simulink model "ME655_Lect09_VL3_Simulink"  (R2021b)
settings: Solver=FixedStepAuto  StartTime=0.0  StopTime=60.0  FixedStep=.003  RelTol=1e-3
values from neighbouring files (symbols this model uses):
  dt_active_control = 10    [ME655_Lect09_VL3_MATLAB.m]
  h = 2.5*N    (= 200)    [ME655_Lect09_VL3_MATLAB.m]
  lambda = .95    (= 0.95)    [ME655_Lect09_VL3_MATLAB.m]
  Lhip_pos0 = Lhip_pos(1)    [ME655_Lect09_VL3_MATLAB.m]
  Lhip_vel0 = Lhip_vel(1)    [ME655_Lect09_VL3_MATLAB.m]
  M = 6    [ME655_Lect09_VL3_MATLAB.m]
  N = 80    [ME655_Lect09_VL3_MATLAB.m]
  nu = .5    (= 0.5)    [ME655_Lect09_VL3_MATLAB.m]
  t_start = 5.0    (= 5)    [ME655_Lect09_VL3_MATLAB.m]
  Tau_h_max = 30    [ME655_Lect09_VL3_MATLAB.m]
undefined symbols (not defined in the file or in its folder): Bh, g, IHC, IRC, Kh, LH, LR, mH, mR, theta_0, theta_d0
settings Model: Creator=Damiano  LastModifiedBy=ilanazane
settings SolverCC: AlgebraicLoopSolver=TrustRegion
settings DataIOCC: ReturnWorkspaceOutputs=off
settings DebuggingCC: SFMachineParentedDataDiag=warning  ArithmeticOperatorsInVariantConditions=warning
settings SFSimCC: SimUseLocalCustomCode=off  CustomCodeUndefinedFunction=UseInterfaceOnly
settings RTWCC: RTWUseLocalCustomCode=off
settings CodeAppCC: StateflowObjectComments=on

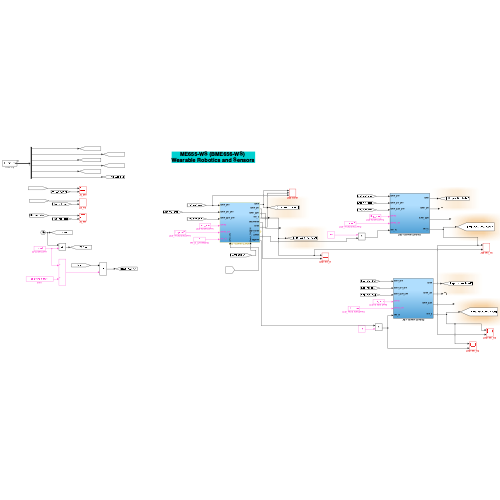
[thumbnail: Simulink's stored preview of the top-level diagram]
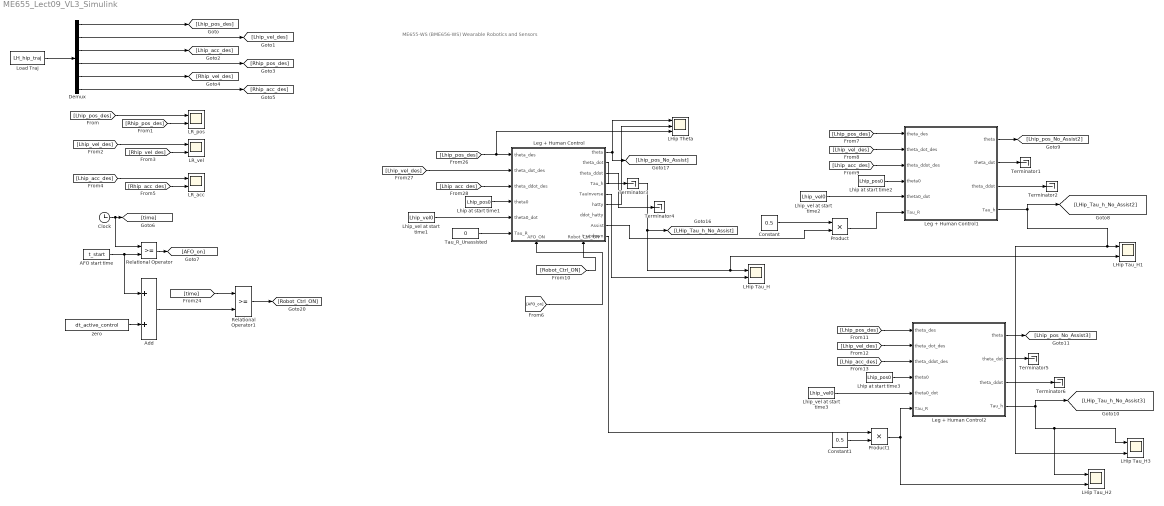
== system ME655_Lect09_VL3_Simulink ==
  note: ME655-WS (BME656-WS)
      | Wearable Robotics and Sensors
  AFO start time : Constant  Value=t_start
  Add : Sum
  Clock : Clock
  Constant : Constant  Value=0.5
  Constant1 : Constant  Value=0.5
  Demux : Demux  Outputs=6
  LHip Tau_H{,1..3} (4 alike) : Scope  NumInputPorts=2
  LHip Theta : Scope  NumInputPorts=3
  "LR_acc " : Scope  NumInputPorts=2
  LR_pos : Scope  NumInputPorts=2
  LR_vel : Scope  NumInputPorts=2
  Leg + Human Control : Subsystem
      settings: PortSchema="{\"entries\":[{\"content\":{\"sides\":[{\"content\":{\"connectorIds\":[\"In1\",\"In2\",\"In3\",\"In4\",\"In5\",\"In6\"]},\"type\":\"ConnectorPlacement.EquallySpacedRectSide\",\"uuid\":\"c89990dd-c7dc-4056-83f4-5e6c1198dd9e\"},{\"content\":{\"connectorIds\":[\"Out1\",\"Out2\",\"Out3\",\"Out4\",\"Out5\",\"Out6\",\"Out7\",\"Out8\",\"Out9\"],\"side\":\"RIGHT\"},\"type\":\"ConnectorPlacement.EquallySpacedRectSide\",\"uuid\":\"97852725-6742-4674-9802-faa7978f5241\"},{\"content\":{\"connectorIds\":[],\"side\":\"TOP\"},\"type\":\"ConnectorPlacement.EquallySpacedRectSide\",\"uuid\":\"eb4c760c-f7ff-400d-9b3e-843f42fb2cfa\"},{\"content\":{\"connectorIds\":[\"In7\",\"In8\"],\"side\":\"BOTTOM\"},\"type\":\"ConnectorPlacement.EquallySpacedRectSide\",\"uuid\":\"cb588bf4-9441-43b4-ae6d-1958c203e45c\"}]},\"type\":\"ConnectorPlacement.EquallySpacedConnector\",\"uuid\":\"443be17b-8f0d-444a-9eaa-10dcd6d34b91\"}],\"packageUris\":[\"http://schema.mathworks.com/mf0/Connector/R2020b\"],\"version\":\"1.0\"}"
  Leg + Human Control1 : Subsystem
  Leg + Human Control2 : Subsystem
  Lhip at start time1 : Constant  Value=Lhip_pos0
  Lhip at start time2 : Constant  Value=Lhip_pos0
  Lhip at start time3 : Constant  Value=Lhip_pos0
  Lhip_vel at start time1 : Constant  Value=Lhip_vel0
  Lhip_vel at start time2 : Constant  Value=Lhip_vel0
  Lhip_vel at start time3 : Constant  Value=Lhip_vel0
  Load Traj : FromWorkspace  VariableName=LH_hip_traj
  Product : Product
  Product1 : Product
  Relational Operator : RelationalOperator  OutDataTypeStr=boolean  RndMeth=Simplest
  Relational Operator1 : RelationalOperator  OutDataTypeStr=boolean  RndMeth=Simplest
  Tau_R_Unassisted : Constant  Value=0
  Terminator{1..6} (6 alike) : Terminator
  zero : Constant  Value=dt_active_control
  wires:
  Load Traj/1 -> Demux/1
  Demux/6 -> [Rhip_acc_des]
  Demux/4 -> [Rhip_pos_des]
  Demux/5 -> [Rhip_vel_des]
  [Lhip_pos_des] -> LR_pos/1
  [Rhip_pos_des] -> LR_pos/2
  [Lhip_vel_des] -> LR_vel/1
  [Rhip_vel_des] -> LR_vel/2
  [Lhip_acc_des] -> "LR_acc "/1
  [Rhip_acc_des] -> "LR_acc "/2
  Clock/1 -> Relational Operator/1, [time]
  Relational Operator/1 -> [AFO_on]
  [time] -> Relational Operator1/1
  AFO start time/1 -> Add/1, Relational Operator/2
  Add/1 -> Relational Operator1/2
  zero/1 -> Add/2
  [Lhip_acc_des] -> Leg + Human Control/3(theta_ddot_des)
  Leg + Human Control/3(theta_ddot) -> Terminator4/1
  Lhip_vel at start time1/1 -> Leg + Human Control/5(theta0_dot)
  Leg + Human Control/2(theta_dot) -> Terminator3/1
  [Lhip_vel_des] -> Leg + Human Control/2(theta_dot_des)
  Lhip at start time1/1 -> Leg + Human Control/4(theta0)
  Leg + Human Control/1(theta) -> [Lhip_pos_No_Assist], LHip Theta/1
  Leg + Human Control/4(Tau_h) -> LHip Tau_H1/2, LHip Tau_H/1, [LHip_Tau_h_No_Assist]
  [Lhip_pos_des] -> Leg + Human Control/1(theta_des), LHip Theta/3
  Relational Operator1/1 -> [Robot_Ctrl_ON]
  Demux/1 -> [Lhip_pos_des]
  Demux/2 -> [Lhip_vel_des]
  Demux/3 -> [Lhip_acc_des]
  Leg + Human Control/5(TauInverse) -> LHip Tau_H/2
  Leg + Human Control/6(hatty) -> LHip Theta/2
  [AFO_on] -> Leg + Human Control/7(AFO_ON)
  Leg + Human Control1/4(Tau_h) -> LHip Tau_H3/2, LHip Tau_H1/1, [LHip_Tau_h_No_Assist2]
  [Lhip_pos_des] -> Leg + Human Control1/1(theta_des)
  Leg + Human Control1/2(theta_dot) -> Terminator1/1
  Lhip_vel at start time2/1 -> Leg + Human Control1/5(theta0_dot)
  [Lhip_acc_des] -> Leg + Human Control1/3(theta_ddot_des)
  Lhip at start time2/1 -> Leg + Human Control1/4(theta0)
  [Lhip_vel_des] -> Leg + Human Control1/2(theta_dot_des)
  Leg + Human Control1/1(theta) -> [Lhip_pos_No_Assist2]
  Leg + Human Control1/3(theta_ddot) -> Terminator2/1
  Tau_R_Unassisted/1 -> Leg + Human Control/6(Tau_R)
  Leg + Human Control/8(Assist) -> Product/2
  Constant/1 -> Product/1
  [Robot_Ctrl_ON] -> Leg + Human Control/8(Robot_Ctrl_ON)
  Product/1 -> Leg + Human Control1/6(Tau_R)
  [Lhip_pos_des] -> Leg + Human Control2/1(theta_des)
  Leg + Human Control2/4(Tau_h) -> LHip Tau_H2/1, LHip Tau_H3/1, [LHip_Tau_h_No_Assist3]
  Leg + Human Control2/1(theta) -> [Lhip_pos_No_Assist3]
  Lhip at start time3/1 -> Leg + Human Control2/4(theta0)
  Lhip_vel at start time3/1 -> Leg + Human Control2/5(theta0_dot)
  [Lhip_acc_des] -> Leg + Human Control2/3(theta_ddot_des)
  Leg + Human Control2/3(theta_ddot) -> Terminator6/1
  [Lhip_vel_des] -> Leg + Human Control2/2(theta_dot_des)
  Leg + Human Control2/2(theta_dot) -> Terminator5/1
  Leg + Human Control/9(t_updown) -> Product1/1
  Constant1/1 -> Product1/2
  Product1/1 -> LHip Tau_H2/2, Leg + Human Control2/6(Tau_R)

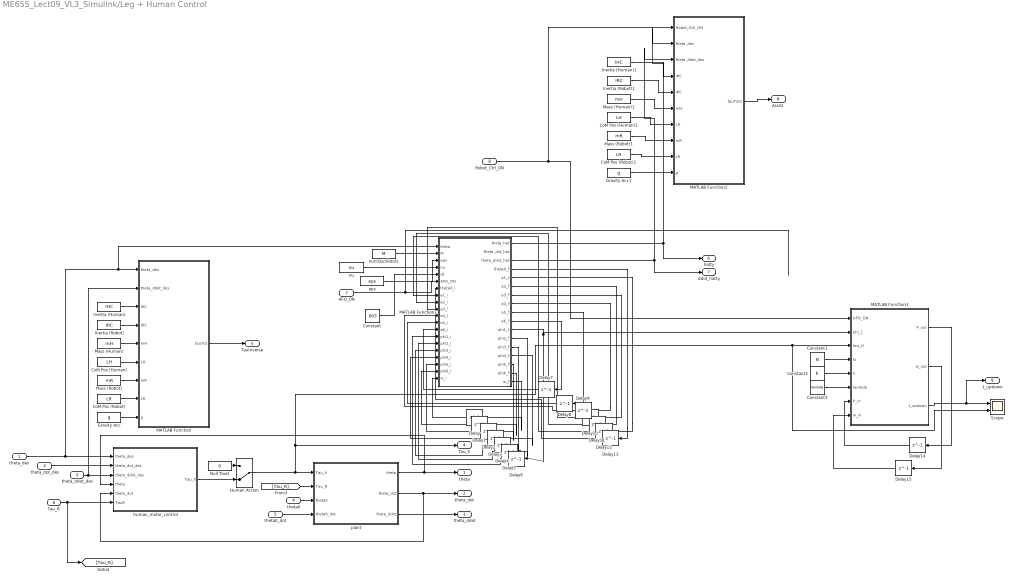
== system ME655_Lect09_VL3_Simulink/Leg + Human Control ==
  theta_des : Inport
  theta_dot_des : Inport  Port=2
  theta_ddot_des : Inport  Port=3
  theta0 : Inport  Port=4
  theta0_dot : Inport  Port=5
  Tau_R : Inport  Port=6
  AFO_ON : Inport  Port=7
  Robot_Ctrl_ON : Inport  Port=8
  CoM Pos (Human) : Constant  Value=LH
  CoM Pos (Human)1 : Constant  Value=LH
  CoM Pos (Robot) : Constant  Value=LR
  CoM Pos (Robot)1 : Constant  Value=LR
  Constant : Constant  Value=.003
  Constant1 : Constant  Value=N
  Constant2 : Constant  Value=h
  Constant3 : Constant  Value=lambda
  Delay{,1..15} (16 alike) : Delay  DelayLength=1  InitialCondition=0
  Gravity Acc : Constant  Value=g
  Gravity Acc1 : Constant  Value=g
  Human Action : ManualSwitch  CurrentSetting=0
  Inertia (Human) : Constant  Value=IHC
  Inertia (Human)1 : Constant  Value=IHC
  Inertia (Robot) : Constant  Value=IRC
  Inertia (Robot)1 : Constant  Value=IRC
  MATLAB Function : MATLAB Function  TreatAsAtomicUnit=on
  MATLAB Function1 : MATLAB Function  TreatAsAtomicUnit=on
  MATLAB Function2 : MATLAB Function  TreatAsAtomicUnit=on
  MATLAB Function3 : MATLAB Function  TreatAsAtomicUnit=on
  Mass (Human) : Constant  Value=mH
  Mass (Human)1 : Constant  Value=mH
  Mass (Robot) : Constant  Value=mR
  Mass (Robot)1 : Constant  Value=mR
  Null TauH : Constant  Value=0
  Scope : Scope  NumInputPorts=2
  eps : Constant  Value=eps
  human_motor_control : Subsystem
  nu : Constant  Value=nu
  numOscillators : Constant  Value=M
  plant : Subsystem
  theta : Outport  PortDimensions=[1,1]  VectorParamsAs1DForOutWhenUnconnected=off
  theta_dot : Outport  Port=2  PortDimensions=[1,1]  VectorParamsAs1DForOutWhenUnconnected=off
  theta_ddot : Outport  Port=3  PortDimensions=[1,1]  VectorParamsAs1DForOutWhenUnconnected=off
  Tau_h : Outport  Port=4  PortDimensions=[1,1]  VectorParamsAs1DForOutWhenUnconnected=off
  TauInverse : Outport  Port=5
  hatty : Outport  Port=6
  ddot_hatty : Outport  Port=7
  Assist : Outport  Port=8
  t_updown : Outport  Port=9
  wires:
  theta_des/1 -> MATLAB Function1/1(theta), MATLAB Function/1(theta_des), human_motor_control/1(theta_des)
  theta_dot_des/1 -> human_motor_control/2(theta_dot_des)
  theta0/1 -> plant/3(theta0)
  theta0_dot/1 -> plant/4(theta0_dot)
  [Tau_R] -> plant/2(Tau_R)
  plant/1(theta) -> theta/1, human_motor_control/4(theta)
  plant/2(theta_dot) -> human_motor_control/5(theta_dot), theta_dot/1
  plant/3(theta_ddot) -> theta_ddot/1
  theta_ddot_des/1 -> MATLAB Function/2(theta_ddot_des), human_motor_control/3(theta_ddot_des)
  human_motor_control/1(Tau_h) -> Human Action/2
  Human Action/1 -> Scope/2, MATLAB Function3/3(tau_H), Tau_h/1, plant/1(Tau_h)
  Null TauH/1 -> Human Action/1
  Tau_R/1 -> [Tau_R], human_motor_control/6(TauR)
  Inertia (Human)/1 -> MATLAB Function/3(IHC)
  Inertia (Robot)/1 -> MATLAB Function/4(IRC)
  Mass (Human)/1 -> MATLAB Function/5(mH)
  CoM Pos (Human)/1 -> MATLAB Function/6(LH)
  Mass (Robot)/1 -> MATLAB Function/7(mR)
  CoM Pos (Robot)/1 -> MATLAB Function/8(LR)
  Gravity Acc/1 -> MATLAB Function/9(g)
  MATLAB Function/1(tauTot) -> TauInverse/1
  numOscillators/1 -> MATLAB Function1/2(M)
  eps/1 -> MATLAB Function1/3(eps)
  nu/1 -> MATLAB Function1/4(nu)
  MATLAB Function1/17(w_f) -> Delay/1
  Delay/1 -> MATLAB Function1/20(w_i)
  MATLAB Function1/16(phi6_f) -> Delay1/1
  Delay1/1 -> MATLAB Function1/19(phi6_i)
  MATLAB Function1/15(phi5_f) -> Delay2/1
  Delay2/1 -> MATLAB Function1/18(phi5_i)
  MATLAB Function1/14(phi4_f) -> Delay3/1
  Delay3/1 -> MATLAB Function1/17(phi4_i)
  MATLAB Function1/13(phi3_f) -> Delay4/1
  Delay4/1 -> MATLAB Function1/16(phi3_i)
  MATLAB Function1/12(phi2_f) -> Delay5/1
  Delay5/1 -> MATLAB Function1/15(phi2_i)
  MATLAB Function1/11(phi1_f) -> Delay6/1, MATLAB Function3/2(phi_1)
  Delay6/1 -> MATLAB Function1/14(phi1_i)
  MATLAB Function1/10(a6_f) -> Delay7/1
  Delay7/1 -> MATLAB Function1/13(a6_i)
  MATLAB Function1/9(a5_f) -> Delay8/1
  Delay8/1 -> MATLAB Function1/12(a5_i)
  MATLAB Function1/8(a4_f) -> Delay9/1
  Delay9/1 -> MATLAB Function1/11(a4_i)
  MATLAB Function1/7(a3_f) -> Delay10/1
  Delay10/1 -> MATLAB Function1/10(a3_i)
  MATLAB Function1/6(a2_f) -> Delay11/1
  Delay11/1 -> MATLAB Function1/9(a2_i)
  MATLAB Function1/5(a1_f) -> Delay12/1
  Delay12/1 -> MATLAB Function1/8(a1_i)
  MATLAB Function1/4(theta0_f) -> Delay13/1
  Delay13/1 -> MATLAB Function1/7(theta0_i)
  Constant/1 -> MATLAB Function1/5(dt)
  MATLAB Function1/1(theta_hat) -> MATLAB Function2/2(theta_des), hatty/1
  AFO_ON/1 -> MATLAB Function1/6(AFO_ON)
  MATLAB Function1/3(theta_ddot_hat) -> ddot_hatty/1, MATLAB Function2/3(theta_ddot_des)
  Inertia (Human)1/1 -> MATLAB Function2/4(IHC)
  Inertia (Robot)1/1 -> MATLAB Function2/5(IRC)
  Mass (Human)1/1 -> MATLAB Function2/6(mH)
  CoM Pos (Human)1/1 -> MATLAB Function2/7(LH)
  Mass (Robot)1/1 -> MATLAB Function2/8(mR)
  CoM Pos (Robot)1/1 -> MATLAB Function2/9(LR)
  Gravity Acc1/1 -> MATLAB Function2/10(g)
  MATLAB Function2/1(tauTot2) -> Assist/1
  Robot_Ctrl_ON/1 -> MATLAB Function3/1(AFO_ON), MATLAB Function2/1(Robot_Ctrl_ON)
  Constant1/1 -> MATLAB Function3/4(N)
  Constant2/1 -> MATLAB Function3/5(h)
  Constant3/1 -> MATLAB Function3/6(lambda)
  Delay14/1 -> MATLAB Function3/7(P_in)
  MATLAB Function3/1(P_out) -> Delay14/1
  MATLAB Function3/2(w_out) -> Delay15/1
  Delay15/1 -> MATLAB Function3/8(w_in)
  MATLAB Function3/3(t_updown) -> t_updown/1, Scope/1

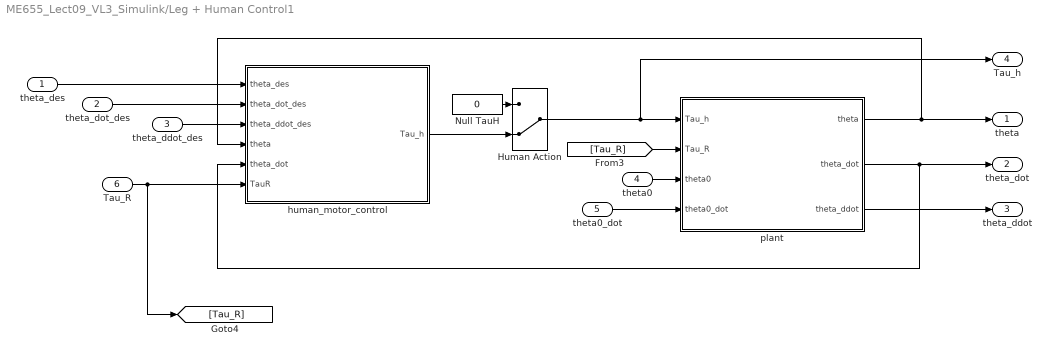
== system ME655_Lect09_VL3_Simulink/Leg + Human Control1 ==
  theta_des : Inport
  theta_dot_des : Inport  Port=2
  theta_ddot_des : Inport  Port=3
  theta0 : Inport  Port=4
  theta0_dot : Inport  Port=5
  Tau_R : Inport  Port=6
  Human Action : ManualSwitch  CurrentSetting=0
  Null TauH : Constant  Value=0
  human_motor_control : Subsystem
  plant : Subsystem
  theta : Outport  PortDimensions=[1,1]  VectorParamsAs1DForOutWhenUnconnected=off
  theta_dot : Outport  Port=2  PortDimensions=[1,1]  VectorParamsAs1DForOutWhenUnconnected=off
  theta_ddot : Outport  Port=3  PortDimensions=[1,1]  VectorParamsAs1DForOutWhenUnconnected=off
  Tau_h : Outport  Port=4  PortDimensions=[1,1]  VectorParamsAs1DForOutWhenUnconnected=off
  wires:
  theta_des/1 -> human_motor_control/1(theta_des)
  theta_dot_des/1 -> human_motor_control/2(theta_dot_des)
  theta0/1 -> plant/3(theta0)
  theta0_dot/1 -> plant/4(theta0_dot)
  [Tau_R] -> plant/2(Tau_R)
  plant/1(theta) -> theta/1, human_motor_control/4(theta)
  plant/2(theta_dot) -> human_motor_control/5(theta_dot), theta_dot/1
  plant/3(theta_ddot) -> theta_ddot/1
  theta_ddot_des/1 -> human_motor_control/3(theta_ddot_des)
  human_motor_control/1(Tau_h) -> Human Action/2
  Human Action/1 -> Tau_h/1, plant/1(Tau_h)
  Null TauH/1 -> Human Action/1
  Tau_R/1 -> [Tau_R], human_motor_control/6(TauR)

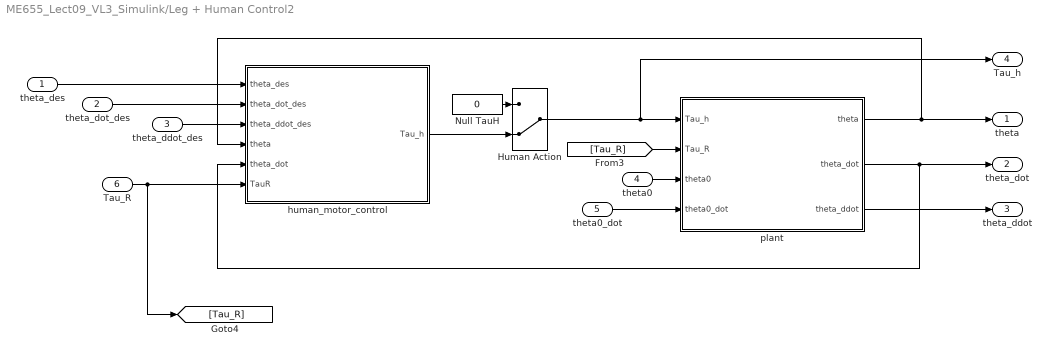
== system ME655_Lect09_VL3_Simulink/Leg + Human Control2 ==
  theta_des : Inport
  theta_dot_des : Inport  Port=2
  theta_ddot_des : Inport  Port=3
  theta0 : Inport  Port=4
  theta0_dot : Inport  Port=5
  Tau_R : Inport  Port=6
  Human Action : ManualSwitch  CurrentSetting=0
  Null TauH : Constant  Value=0
  human_motor_control : Subsystem
  plant : Subsystem
  theta : Outport  PortDimensions=[1,1]  VectorParamsAs1DForOutWhenUnconnected=off
  theta_dot : Outport  Port=2  PortDimensions=[1,1]  VectorParamsAs1DForOutWhenUnconnected=off
  theta_ddot : Outport  Port=3  PortDimensions=[1,1]  VectorParamsAs1DForOutWhenUnconnected=off
  Tau_h : Outport  Port=4  PortDimensions=[1,1]  VectorParamsAs1DForOutWhenUnconnected=off
  wires:
  theta_des/1 -> human_motor_control/1(theta_des)
  theta_dot_des/1 -> human_motor_control/2(theta_dot_des)
  theta0/1 -> plant/3(theta0)
  theta0_dot/1 -> plant/4(theta0_dot)
  [Tau_R] -> plant/2(Tau_R)
  plant/1(theta) -> theta/1, human_motor_control/4(theta)
  plant/2(theta_dot) -> human_motor_control/5(theta_dot), theta_dot/1
  plant/3(theta_ddot) -> theta_ddot/1
  theta_ddot_des/1 -> human_motor_control/3(theta_ddot_des)
  human_motor_control/1(Tau_h) -> Human Action/2
  Human Action/1 -> Tau_h/1, plant/1(Tau_h)
  Null TauH/1 -> Human Action/1
  Tau_R/1 -> [Tau_R], human_motor_control/6(TauR)

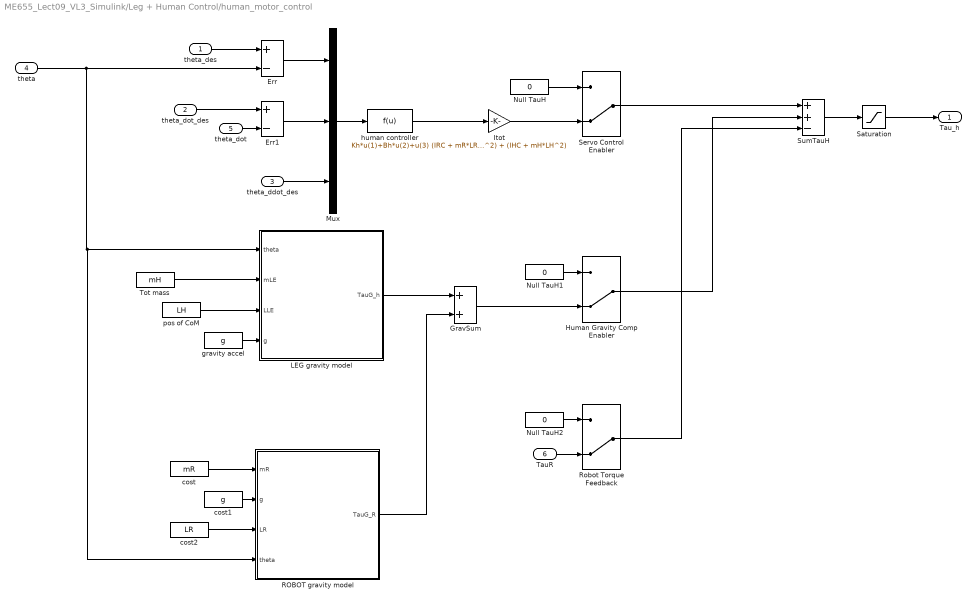
== system ME655_Lect09_VL3_Simulink/Leg + Human Control/human_motor_control ==
  theta_des : Inport
  theta_dot_des : Inport  Port=2
  theta_ddot_des : Inport  Port=3
  theta : Inport  Port=4
  theta_dot : Inport  Port=5
  TauR : Inport  Port=6
  Err : Sum  Inputs=+-
  Err1 : Sum  Inputs=+-
  GravSum : Sum
  Human Gravity Comp Enabler : ManualSwitch  CurrentSetting=0
  Itot : Gain  Gain=(IRC + mR*LR^2) + (IHC + mH*LH^2)
  LEG gravity model : MATLAB Function  TreatAsAtomicUnit=on
  Mux : Mux  Inputs=3
  Null TauH : Constant  Value=0
  Null TauH1 : Constant  Value=0
  Null TauH2 : Constant  Value=0
  ROBOT gravity model : MATLAB Function  TreatAsAtomicUnit=on
  Robot Torque Feedback : ManualSwitch  CurrentSetting=0
  Saturation : Saturate  UpperLimit=Tau_h_max  LowerLimit=-Tau_h_max
  Servo Control Enabler : ManualSwitch  CurrentSetting=0
  SumTauH : Sum  Inputs=++-
  Tot mass : Constant  Value=mH
  cost : Constant  Value=mR
  cost1 : Constant  Value=g
  cost2 : Constant  Value=LR
  gravity accel : Constant  Value=g
  human controller : Fcn  Expr=Kh*u(1)+Bh*u(2)+u(3)
  pos of CoM : Constant  Value=LH
  Tau_h : Outport  PortDimensions=[1,1]  VectorParamsAs1DForOutWhenUnconnected=off
  wires:
  theta_des/1 -> Err/1
  theta_dot_des/1 -> Err1/1
  theta_dot/1 -> Err1/2
  Err/1 -> Mux/1
  Err1/1 -> Mux/2
  Mux/1 -> human controller/1
  theta_ddot_des/1 -> Mux/3
  gravity accel/1 -> LEG gravity model/4(g)
  Tot mass/1 -> LEG gravity model/2(mLE)
  pos of CoM/1 -> LEG gravity model/3(LLE)
  Null TauH/1 -> Servo Control Enabler/1
  Null TauH1/1 -> Human Gravity Comp Enabler/1
  Human Gravity Comp Enabler/1 -> SumTauH/2
  SumTauH/1 -> Saturation/1
  human controller/1 -> Itot/1
  Servo Control Enabler/1 -> SumTauH/1
  Saturation/1 -> Tau_h/1
  Itot/1 -> Servo Control Enabler/2
  Null TauH2/1 -> Robot Torque Feedback/1
  TauR/1 -> Robot Torque Feedback/2
  Robot Torque Feedback/1 -> SumTauH/3
  theta/1 -> ROBOT gravity model/4(theta), LEG gravity model/1(theta), Err/2
  ROBOT gravity model/1(TauG_R) -> GravSum/2
  cost2/1 -> ROBOT gravity model/3(LR)
  cost/1 -> ROBOT gravity model/1(mR)
  cost1/1 -> ROBOT gravity model/2(g)
  LEG gravity model/1(TauG_h) -> GravSum/1
  GravSum/1 -> Human Gravity Comp Enabler/2

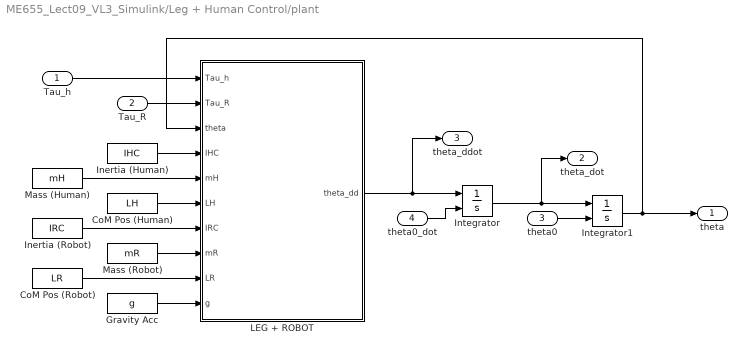
== system ME655_Lect09_VL3_Simulink/Leg + Human Control/plant ==
  Tau_h : Inport
  Tau_R : Inport  Port=2
  theta0 : Inport  Port=3
  theta0_dot : Inport  Port=4
  CoM Pos (Human) : Constant  Value=LH
  CoM Pos (Robot) : Constant  Value=LR
  Gravity Acc : Constant  Value=g
  Inertia (Human) : Constant  Value=IHC  VectorParams1D=off
  Inertia (Robot) : Constant  Value=IRC
  Integrator : Integrator  InitialConditionSource=external  InitialCondition=theta_d0
  Integrator1 : Integrator  InitialConditionSource=external  InitialCondition=theta_0
  LEG + ROBOT : MATLAB Function  TreatAsAtomicUnit=on
  Mass (Human) : Constant  Value=mH
  Mass (Robot) : Constant  Value=mR
  theta : Outport  PortDimensions=[1,1]  VectorParamsAs1DForOutWhenUnconnected=off
  theta_dot : Outport  Port=2  PortDimensions=[1,1]  VectorParamsAs1DForOutWhenUnconnected=off
  theta_ddot : Outport  Port=3  PortDimensions=[1,1]  VectorParamsAs1DForOutWhenUnconnected=off
  wires:
  Tau_h/1 -> LEG + ROBOT/1(Tau_h)
  Tau_R/1 -> LEG + ROBOT/2(Tau_R)
  LEG + ROBOT/1(theta_dd) -> theta_ddot/1, Integrator/1
  Integrator/1 -> theta_dot/1, Integrator1/1
  theta0_dot/1 -> Integrator/2
  theta0/1 -> Integrator1/2
  Integrator1/1 -> LEG + ROBOT/3(theta), theta/1
  Inertia (Human)/1 -> LEG + ROBOT/4(IHC)
  Mass (Human)/1 -> LEG + ROBOT/5(mH)
  CoM Pos (Human)/1 -> LEG + ROBOT/6(LH)
  Gravity Acc/1 -> LEG + ROBOT/10(g)
  Mass (Robot)/1 -> LEG + ROBOT/8(mR)
  CoM Pos (Robot)/1 -> LEG + ROBOT/9(LR)
  Inertia (Robot)/1 -> LEG + ROBOT/7(IRC)

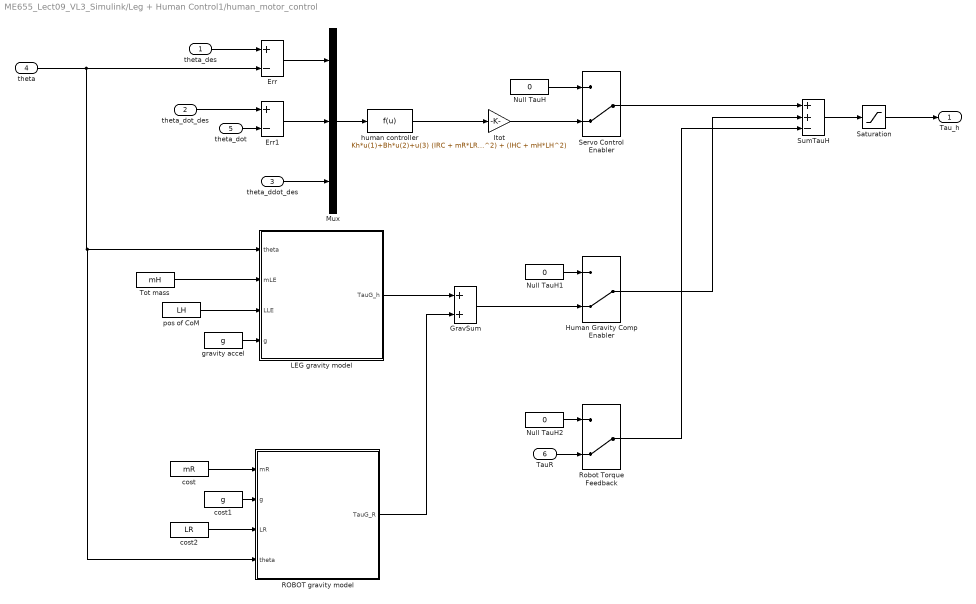
== system ME655_Lect09_VL3_Simulink/Leg + Human Control1/human_motor_control ==
  theta_des : Inport
  theta_dot_des : Inport  Port=2
  theta_ddot_des : Inport  Port=3
  theta : Inport  Port=4
  theta_dot : Inport  Port=5
  TauR : Inport  Port=6
  Err : Sum  Inputs=+-
  Err1 : Sum  Inputs=+-
  GravSum : Sum
  Human Gravity Comp Enabler : ManualSwitch  CurrentSetting=0
  Itot : Gain  Gain=(IRC + mR*LR^2) + (IHC + mH*LH^2)
  LEG gravity model : MATLAB Function  TreatAsAtomicUnit=on
  Mux : Mux  Inputs=3
  Null TauH : Constant  Value=0
  Null TauH1 : Constant  Value=0
  Null TauH2 : Constant  Value=0
  ROBOT gravity model : MATLAB Function  TreatAsAtomicUnit=on
  Robot Torque Feedback : ManualSwitch  CurrentSetting=0
  Saturation : Saturate  UpperLimit=Tau_h_max  LowerLimit=-Tau_h_max
  Servo Control Enabler : ManualSwitch  CurrentSetting=0
  SumTauH : Sum  Inputs=++-
  Tot mass : Constant  Value=mH
  cost : Constant  Value=mR
  cost1 : Constant  Value=g
  cost2 : Constant  Value=LR
  gravity accel : Constant  Value=g
  human controller : Fcn  Expr=Kh*u(1)+Bh*u(2)+u(3)
  pos of CoM : Constant  Value=LH
  Tau_h : Outport  PortDimensions=[1,1]  VectorParamsAs1DForOutWhenUnconnected=off
  wires:
  theta_des/1 -> Err/1
  theta_dot_des/1 -> Err1/1
  theta_dot/1 -> Err1/2
  Err/1 -> Mux/1
  Err1/1 -> Mux/2
  Mux/1 -> human controller/1
  theta_ddot_des/1 -> Mux/3
  gravity accel/1 -> LEG gravity model/4(g)
  Tot mass/1 -> LEG gravity model/2(mLE)
  pos of CoM/1 -> LEG gravity model/3(LLE)
  Null TauH/1 -> Servo Control Enabler/1
  Null TauH1/1 -> Human Gravity Comp Enabler/1
  Human Gravity Comp Enabler/1 -> SumTauH/2
  SumTauH/1 -> Saturation/1
  human controller/1 -> Itot/1
  Servo Control Enabler/1 -> SumTauH/1
  Saturation/1 -> Tau_h/1
  Itot/1 -> Servo Control Enabler/2
  Null TauH2/1 -> Robot Torque Feedback/1
  TauR/1 -> Robot Torque Feedback/2
  Robot Torque Feedback/1 -> SumTauH/3
  theta/1 -> ROBOT gravity model/4(theta), LEG gravity model/1(theta), Err/2
  ROBOT gravity model/1(TauG_R) -> GravSum/2
  cost2/1 -> ROBOT gravity model/3(LR)
  cost/1 -> ROBOT gravity model/1(mR)
  cost1/1 -> ROBOT gravity model/2(g)
  LEG gravity model/1(TauG_h) -> GravSum/1
  GravSum/1 -> Human Gravity Comp Enabler/2

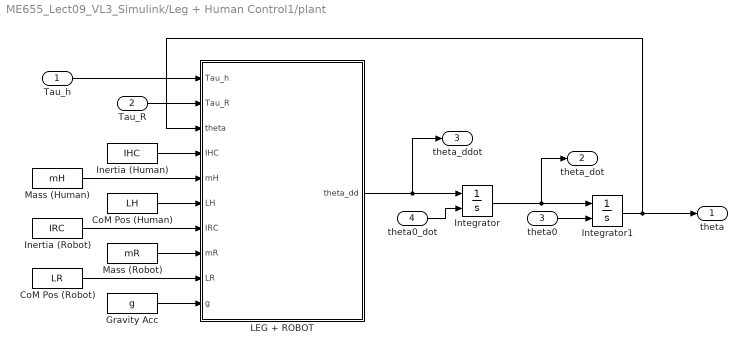
== system ME655_Lect09_VL3_Simulink/Leg + Human Control1/plant ==
  Tau_h : Inport
  Tau_R : Inport  Port=2
  theta0 : Inport  Port=3
  theta0_dot : Inport  Port=4
  CoM Pos (Human) : Constant  Value=LH
  CoM Pos (Robot) : Constant  Value=LR
  Gravity Acc : Constant  Value=g
  Inertia (Human) : Constant  Value=IHC  VectorParams1D=off
  Inertia (Robot) : Constant  Value=IRC
  Integrator : Integrator  InitialConditionSource=external  InitialCondition=theta_d0
  Integrator1 : Integrator  InitialConditionSource=external  InitialCondition=theta_0
  LEG + ROBOT : MATLAB Function  TreatAsAtomicUnit=on
  Mass (Human) : Constant  Value=mH
  Mass (Robot) : Constant  Value=mR
  theta : Outport  PortDimensions=[1,1]  VectorParamsAs1DForOutWhenUnconnected=off
  theta_dot : Outport  Port=2  PortDimensions=[1,1]  VectorParamsAs1DForOutWhenUnconnected=off
  theta_ddot : Outport  Port=3  PortDimensions=[1,1]  VectorParamsAs1DForOutWhenUnconnected=off
  wires:
  Tau_h/1 -> LEG + ROBOT/1(Tau_h)
  Tau_R/1 -> LEG + ROBOT/2(Tau_R)
  LEG + ROBOT/1(theta_dd) -> theta_ddot/1, Integrator/1
  Integrator/1 -> theta_dot/1, Integrator1/1
  theta0_dot/1 -> Integrator/2
  theta0/1 -> Integrator1/2
  Integrator1/1 -> LEG + ROBOT/3(theta), theta/1
  Inertia (Human)/1 -> LEG + ROBOT/4(IHC)
  Mass (Human)/1 -> LEG + ROBOT/5(mH)
  CoM Pos (Human)/1 -> LEG + ROBOT/6(LH)
  Gravity Acc/1 -> LEG + ROBOT/10(g)
  Mass (Robot)/1 -> LEG + ROBOT/8(mR)
  CoM Pos (Robot)/1 -> LEG + ROBOT/9(LR)
  Inertia (Robot)/1 -> LEG + ROBOT/7(IRC)

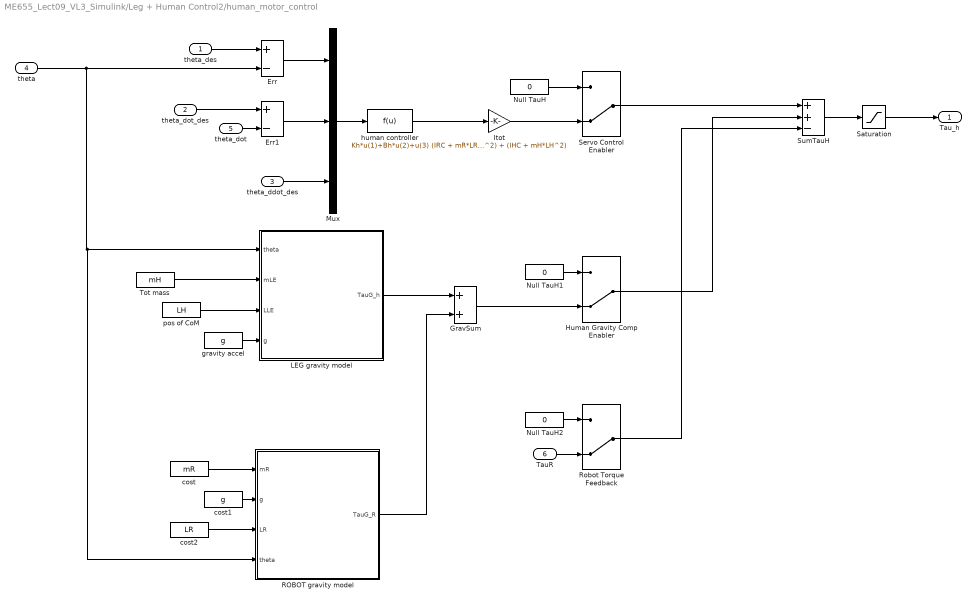
== system ME655_Lect09_VL3_Simulink/Leg + Human Control2/human_motor_control ==
  theta_des : Inport
  theta_dot_des : Inport  Port=2
  theta_ddot_des : Inport  Port=3
  theta : Inport  Port=4
  theta_dot : Inport  Port=5
  TauR : Inport  Port=6
  Err : Sum  Inputs=+-
  Err1 : Sum  Inputs=+-
  GravSum : Sum
  Human Gravity Comp Enabler : ManualSwitch  CurrentSetting=0
  Itot : Gain  Gain=(IRC + mR*LR^2) + (IHC + mH*LH^2)
  LEG gravity model : MATLAB Function  TreatAsAtomicUnit=on
  Mux : Mux  Inputs=3
  Null TauH : Constant  Value=0
  Null TauH1 : Constant  Value=0
  Null TauH2 : Constant  Value=0
  ROBOT gravity model : MATLAB Function  TreatAsAtomicUnit=on
  Robot Torque Feedback : ManualSwitch  CurrentSetting=0
  Saturation : Saturate  UpperLimit=Tau_h_max  LowerLimit=-Tau_h_max
  Servo Control Enabler : ManualSwitch  CurrentSetting=0
  SumTauH : Sum  Inputs=++-
  Tot mass : Constant  Value=mH
  cost : Constant  Value=mR
  cost1 : Constant  Value=g
  cost2 : Constant  Value=LR
  gravity accel : Constant  Value=g
  human controller : Fcn  Expr=Kh*u(1)+Bh*u(2)+u(3)
  pos of CoM : Constant  Value=LH
  Tau_h : Outport  PortDimensions=[1,1]  VectorParamsAs1DForOutWhenUnconnected=off
  wires:
  theta_des/1 -> Err/1
  theta_dot_des/1 -> Err1/1
  theta_dot/1 -> Err1/2
  Err/1 -> Mux/1
  Err1/1 -> Mux/2
  Mux/1 -> human controller/1
  theta_ddot_des/1 -> Mux/3
  gravity accel/1 -> LEG gravity model/4(g)
  Tot mass/1 -> LEG gravity model/2(mLE)
  pos of CoM/1 -> LEG gravity model/3(LLE)
  Null TauH/1 -> Servo Control Enabler/1
  Null TauH1/1 -> Human Gravity Comp Enabler/1
  Human Gravity Comp Enabler/1 -> SumTauH/2
  SumTauH/1 -> Saturation/1
  human controller/1 -> Itot/1
  Servo Control Enabler/1 -> SumTauH/1
  Saturation/1 -> Tau_h/1
  Itot/1 -> Servo Control Enabler/2
  Null TauH2/1 -> Robot Torque Feedback/1
  TauR/1 -> Robot Torque Feedback/2
  Robot Torque Feedback/1 -> SumTauH/3
  theta/1 -> ROBOT gravity model/4(theta), LEG gravity model/1(theta), Err/2
  ROBOT gravity model/1(TauG_R) -> GravSum/2
  cost2/1 -> ROBOT gravity model/3(LR)
  cost/1 -> ROBOT gravity model/1(mR)
  cost1/1 -> ROBOT gravity model/2(g)
  LEG gravity model/1(TauG_h) -> GravSum/1
  GravSum/1 -> Human Gravity Comp Enabler/2

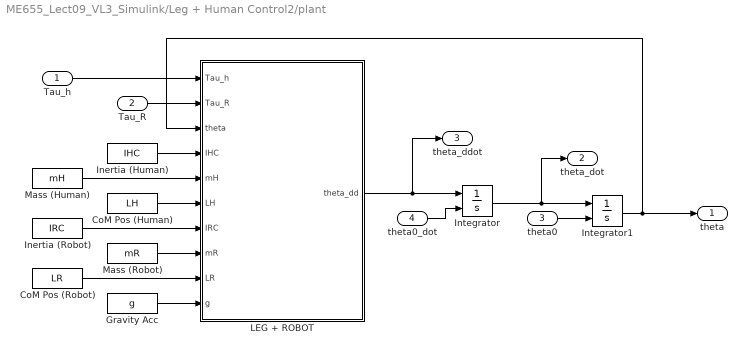
== system ME655_Lect09_VL3_Simulink/Leg + Human Control2/plant ==
  Tau_h : Inport
  Tau_R : Inport  Port=2
  theta0 : Inport  Port=3
  theta0_dot : Inport  Port=4
  CoM Pos (Human) : Constant  Value=LH
  CoM Pos (Robot) : Constant  Value=LR
  Gravity Acc : Constant  Value=g
  Inertia (Human) : Constant  Value=IHC  VectorParams1D=off
  Inertia (Robot) : Constant  Value=IRC
  Integrator : Integrator  InitialConditionSource=external  InitialCondition=theta_d0
  Integrator1 : Integrator  InitialConditionSource=external  InitialCondition=theta_0
  LEG + ROBOT : MATLAB Function  TreatAsAtomicUnit=on
  Mass (Human) : Constant  Value=mH
  Mass (Robot) : Constant  Value=mR
  theta : Outport  PortDimensions=[1,1]  VectorParamsAs1DForOutWhenUnconnected=off
  theta_dot : Outport  Port=2  PortDimensions=[1,1]  VectorParamsAs1DForOutWhenUnconnected=off
  theta_ddot : Outport  Port=3  PortDimensions=[1,1]  VectorParamsAs1DForOutWhenUnconnected=off
  wires:
  Tau_h/1 -> LEG + ROBOT/1(Tau_h)
  Tau_R/1 -> LEG + ROBOT/2(Tau_R)
  LEG + ROBOT/1(theta_dd) -> theta_ddot/1, Integrator/1
  Integrator/1 -> theta_dot/1, Integrator1/1
  theta0_dot/1 -> Integrator/2
  theta0/1 -> Integrator1/2
  Integrator1/1 -> LEG + ROBOT/3(theta), theta/1
  Inertia (Human)/1 -> LEG + ROBOT/4(IHC)
  Mass (Human)/1 -> LEG + ROBOT/5(mH)
  CoM Pos (Human)/1 -> LEG + ROBOT/6(LH)
  Gravity Acc/1 -> LEG + ROBOT/10(g)
  Mass (Robot)/1 -> LEG + ROBOT/8(mR)
  CoM Pos (Robot)/1 -> LEG + ROBOT/9(LR)
  Inertia (Robot)/1 -> LEG + ROBOT/7(IRC)

== matlab function ME655_Lect09_VL3_Simulink/Leg + Human Control/MATLAB Function2 ==
  data: Robot_Ctrl_ON input; theta_des input; tauTot2 output; theta_ddot_des input; IHC input; IRC input; mH input; LH input; mR input; LR input; g input
function tauTot2 = InverseDyn(Robot_Ctrl_ON, theta_des,theta_ddot_des,IHC,IRC,mH,LH,mR,LR,g)

if Robot_Ctrl_ON == 0
    tauTot2 = 0;
    return
else
    tauTot2 = (IHC + IRC + mH*LH^2 +mR*LR^2)*theta_ddot_des + (mH*LH+mR*LR)*g*sin(theta_des);

end

== matlab function ME655_Lect09_VL3_Simulink/Leg + Human Control/MATLAB Function3 ==
  data: AFO_ON input; phi_1 input; tau_H input; N input; h input; lambda input; P_out output; P_in input; w_in input; w_out output; t_updown output
function [P_out, w_out, t_updown]  = fcn(AFO_ON,phi_1, tau_H, N, h, lambda, P_in, w_in)

if AFO_ON == 0
    P_in = ones(1,80);
    w_in = zeros(1,80);
    P_out = real(P_in);
    w_out = w_in;
    t_updown = 0;
else
    P_in = P_in;
    P_out = zeros(1,80);
    w_out = zeros(1,80);
    psi = zeros(1,80);
    e = zeros(1,80);
    
    for c = 1:80
        e(c) = tau_H - w_in(c);
        psi(c) = exp(h*cos(phi_1 - (2*pi*c/80)) - h);
        
        P_out(c) = (P_in(c) - ( P_in(c)^2 / ((lambda/psi(c) + P_in(c)) ) ) ) / lambda;
        
        

        w_out(c) = w_in(c) + psi(c)*real(P_out(c))*e(c);
    end
    t_updown = dot(psi, w_in)/sum(psi);
end

== matlab function ME655_Lect09_VL3_Simulink/Leg + Human Control2/human_motor_control/LEG gravity model ==
  data: theta input; mLE input; LLE input; TauG_h output; g input
function TauG_h   = HumanLegGravModel(theta,mLE,LLE,g)
% human gravity compensation term
TauG_h=mLE*g*LLE*sin(theta);

end

== matlab function ME655_Lect09_VL3_Simulink/Leg + Human Control2/human_motor_control/ROBOT gravity model ==
  data: mR input; g input; LR input; theta input; TauG_R output
function TauG_R  = RobotGravModel(mR,g,LR,theta)

TauG_R=mR*g*LR*sin(theta);
% TauG_h=mLE*g*LLE*sin(theta);

end

== matlab function ME655_Lect09_VL3_Simulink/Leg + Human Control1/human_motor_control/LEG gravity model ==
  data: theta input; mLE input; LLE input; TauG_h output; g input
function TauG_h   = HumanLegGravModel(theta,mLE,LLE,g)
% human gravity compensation term
TauG_h=mLE*g*LLE*sin(theta);

end

== matlab function ME655_Lect09_VL3_Simulink/Leg + Human Control1/human_motor_control/ROBOT gravity model ==
  data: mR input; g input; LR input; theta input; TauG_R output
function TauG_R  = RobotGravModel(mR,g,LR,theta)

TauG_R=mR*g*LR*sin(theta);
% TauG_h=mLE*g*LLE*sin(theta);

end

== matlab function ME655_Lect09_VL3_Simulink/Leg + Human Control/human_motor_control/LEG gravity model ==
  data: theta input; mLE input; LLE input; TauG_h output; g input
function TauG_h   = HumanLegGravModel(theta,mLE,LLE,g)
% human gravity compensation term
TauG_h=mLE*g*LLE*sin(theta);

end

== matlab function ME655_Lect09_VL3_Simulink/Leg + Human Control1/plant/LEG + ROBOT ==
  data: Tau_h input; Tau_R input; theta input; theta_dd output; IHC input; mH input; LH input; IRC input; mR input; LR input; g input
function theta_dd = LegRobotModel(Tau_h, Tau_R, theta, IHC, mH, LH, IRC, mR, LR, g)
theta_dd = 1/((IRC + mR*LR^2)+(IHC + mH*LH^2)) * (Tau_h-mH*g*LH*sin(theta) + Tau_R-mR*g*LR*sin(theta));
end

== matlab function ME655_Lect09_VL3_Simulink/Leg + Human Control2/plant/LEG + ROBOT ==
  data: Tau_h input; Tau_R input; theta input; theta_dd output; IHC input; mH input; LH input; IRC input; mR input; LR input; g input
function theta_dd = LegRobotModel(Tau_h, Tau_R, theta, IHC, mH, LH, IRC, mR, LR, g)
theta_dd = 1/((IRC + mR*LR^2)+(IHC + mH*LH^2)) * (Tau_h-mH*g*LH*sin(theta) + Tau_R-mR*g*LR*sin(theta));
end

== matlab function ME655_Lect09_VL3_Simulink/Leg + Human Control/human_motor_control/ROBOT gravity model ==
  data: mR input; g input; LR input; theta input; TauG_R output
function TauG_R  = RobotGravModel(mR,g,LR,theta)

TauG_R=mR*g*LR*sin(theta);
% TauG_h=mLE*g*LLE*sin(theta);

end

== matlab function ME655_Lect09_VL3_Simulink/Leg + Human Control/plant/LEG + ROBOT ==
  data: Tau_h input; Tau_R input; theta input; theta_dd output; IHC input; mH input; LH input; IRC input; mR input; LR input; g input
function theta_dd = LegRobotModel(Tau_h, Tau_R, theta, IHC, mH, LH, IRC, mR, LR, g)
theta_dd = 1/((IRC + mR*LR^2)+(IHC + mH*LH^2)) * (Tau_h-mH*g*LH*sin(theta) + Tau_R-mR*g*LR*sin(theta));
end

== matlab function ME655_Lect09_VL3_Simulink/Leg + Human Control/MATLAB Function1 ==
  data: theta_hat output; theta input; theta_dot_hat output; theta_ddot_hat output; theta0_f output; M input; eps input; nu input; dt input; AFO_ON input; theta0_i input; a1_i input; a2_i input; a3_i input; a4_i input; a5_i input; a6_i input; phi1_i input; phi2_i input; phi3_i input; phi4_i input; phi5_i input; phi6_i input; w_i input; a1_f output; a2_f output; a3_f output; a4_f output; a5_f output; a6_f output; phi1_f output; phi2_f output; phi3_f output; phi4_f output; phi5_f output; phi6_f output; w_f output
function [theta_hat,theta_dot_hat,theta_ddot_hat, theta0_f, a1_f, a2_f, a3_f, a4_f, a5_f, a6_f, phi1_f, phi2_f, phi3_f, phi4_f, phi5_f, phi6_f, w_f] = AFO(theta,M,eps,nu,dt,AFO_ON, theta0_i, a1_i, a2_i, a3_i, a4_i, a5_i, a6_i, phi1_i, phi2_i, phi3_i, phi4_i, phi5_i, phi6_i, w_i)

if AFO_ON == 0
    theta_hat = 0;
    theta_dot_hat = 0;
    theta_ddot_hat = 0;
    theta0_f = 0;
    a1_f = 0;
    a2_f = 0;
    a3_f = 0;
    a4_f = 0;
    a5_f = 0;
    a6_f = 0;
    phi1_f = 0;
    phi2_f = 0;
    phi3_f = 0;
    phi4_f = 0;
    phi5_f = 0;
    phi6_f = 0;
    w_f = 0;

    return

else

    if phi1_i == 0 & phi2_i == 0 & phi3_i == 0 & phi4_i == 0 & phi5_i == 0 & phi6_i == 0 & w_i == 0
        phi1_i = pi/2;
        phi2_i = pi/2;
        phi3_i = pi/2;
        phi4_i = pi/2;
        phi5_i = pi/2;
        phi6_i = pi/2;
        w_i = 3*pi/2;
    end
    
    F = theta - theta0_i - a1_i*sin(phi1_i)- a2_i*sin(phi2_i)- a3_i*sin(phi3_i)- a4_i*sin(phi4_i)- a5_i*sin(phi5_i)- a6_i*sin(phi6_i);
    
    phi1_f = mod(phi1_i + dt*(1*w_i+eps*F*cos(phi1_i)), 2*pi);
    phi2_f = mod(phi2_i + dt*(2*w_i+eps*F*cos(phi2_i)), 2*pi);
    phi3_f = mod(phi3_i + dt*(3*w_i+eps*F*cos(phi3_i)), 2*pi);
    phi4_f = mod(phi4_i + dt*(4*w_i+eps*F*cos(phi4_i)), 2*pi);
    phi5_f = mod(phi5_i + dt*(5*w_i+eps*F*cos(phi5_i)), 2*pi);
    phi6_f = mod(phi6_i + dt*(6*w_i+eps*F*cos(phi6_i)), 2*pi);
    
    theta0_f = theta0_i + dt*nu*F;
    
    a1_f = a1_i + dt*nu*F*sin(phi1_i);
    a2_f = a2_i + dt*nu*F*sin(phi2_i);
    a3_f = a3_i + dt*nu*F*sin(phi3_i);
    a4_f = a4_i + dt*nu*F*sin(phi4_i);
    a5_f = a5_i + dt*nu*F*sin(phi5_i);
    a6_f = a6_i + dt*nu*F*sin(phi6_i);
    
    
    w_f = w_i + dt*eps*F*cos(phi1_i);
    
    theta_hat = theta0_f + a1_f*sin(phi1_f)+ a2_f*sin(phi2_f)+ a3_f*sin(phi3_f)+ a4_f*sin(phi4_f)+ a5_f*sin(phi5_f)+ a6_f*sin(phi6_f);
    theta_dot_hat = 0;
    theta_ddot_hat = -1*w_f^2*a1_f*sin(phi1_f)- 2*w_f^2*a2_f*sin(phi2_f)- 3*w_f^2*a3_f*sin(phi3_f)- 4*w_f^2*a4_f*sin(phi4_f)- 5*w_f^2*a5_f*sin(phi5_f)- 6*w_f^2*a6_f*sin(phi6_f);

end

== matlab function ME655_Lect09_VL3_Simulink/Leg + Human Control/MATLAB Function ==
  data: theta_des input; tauTot output; theta_ddot_des input; IHC input; IRC input; mH input; LH input; mR input; LR input; g input
function tauTot = InverseDyn(theta_des,theta_ddot_des,IHC,IRC,mH,LH,mR,LR,g)

tauTot = (IHC + IRC + mH*LH^2 +mR*LR^2)*theta_ddot_des + (mH*LH+mR*LR)*g*sin(theta_des);

end
